simulink model "Copy_of_HIL_Serial"  (R2020a)
settings: Solver=ode4  StartTime=0.0  StopTime=inf  FixedStep=0.01  RelTol=1e-3  EnableMultiTasking=on
values from neighbouring files (symbols this model uses):
  Ue = [0.0416; -0.0703; 0; 0]    [equilibrium.m]    (also in start.m = [0.0416; -0.0703;      0;      0])
undefined symbols (not defined in the file or in its folder): LF, serial
libraries: instrumentlib x3
settings Model: PauseTimes=29  Creator=Marcelo Henrique  LastModifiedBy=waldene
settings SolverCC: AlgebraicLoopSolver=LineSearch
settings DataIOCC: LimitDataPoints=on  SaveFormat=Array  ReturnWorkspaceOutputs=off
settings OptimizationCC: LifeSpan=inf
settings DebuggingCC: AlgebraicLoopMsg=none  UnderspecifiedInitializationDetection=Classic  MergeDetectMultiDrivingBlocksExec=none  StateNameClashWarn=warning  SFUnexpectedBacktrackingDiag=warning  SFNoUnconditionalDefaultTransitionDiag=warning  ArithmeticOperatorsInVariantConditions=warning
settings HardwareCC: ProdBitPerPointer=32  ProdBitPerSizeT=32  ProdBitPerPtrDiffT=32  ProdLargestAtomicFloat=None  ProdIntDivRoundTo=Undefined  ProdEndianess=Unspecified  ProdWordSize=32  ProdHWDeviceType=32-bit Generic
settings ModelReferenceCC: PropagateSignalLabelsOutOfModel=off
settings SFSimCC: SimUseLocalCustomCode=off  CustomCodeUndefinedFunction=UseInterfaceOnly
settings RTWCC: RTWUseLocalCustomCode=off
settings CodeAppCC: StateflowObjectComments=on
settings GRTTargetCC: TargetLangStandard=C89/C90 (ANSI)
settings ConfigComp: CovMetricSettings=dw  CovHtmlReporting=on  CovSaveCumulativeToWorkspaceVar=on  CovSaveSingleToWorkspaceVar=on  CovExternalEMLEnable=off

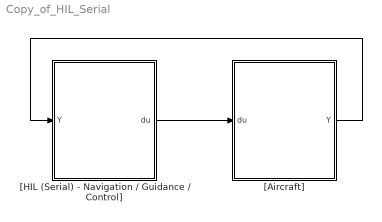
== system Copy_of_HIL_Serial ==
  "[Aircraft]" : Subsystem
  "[HIL (Serial) - Navigation / Guidance / Control]" : Subsystem
  wires:
  "[Aircraft]"/1(Y) -> "[HIL (Serial) - Navigation / Guidance / Control]"/1(Y)
  "[HIL (Serial) - Navigation / Guidance / Control]"/1(du) -> "[Aircraft]"/1(du)

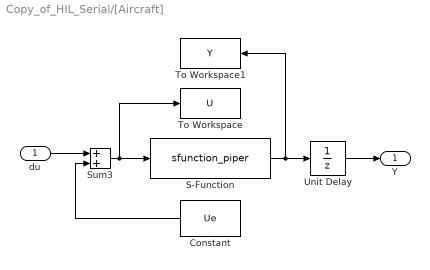
== system Copy_of_HIL_Serial/[Aircraft] ==
  du : Inport
  Constant : Constant  Value=Ue
  S-Function : S-Function  FunctionName=sfunction_piper  Parameters=par_gen,par_aero,par_prop, Xe  SFunctionDeploymentMode=off  EnableBusSupport=off
  Sum3 : Sum
  To Workspace : ToWorkspace  VariableName=U  SaveFormat=Timeseries  SampleTime=-1
  To Workspace1 : ToWorkspace  VariableName=Y  SaveFormat=Timeseries  SampleTime=-1
  Unit Delay : UnitDelay  SampleTime=-1  HasFrameUpgradeWarning=on
  Y : Outport
  wires:
  du/1 -> Sum3/1
  S-Function/1 -> To Workspace1/1, Unit Delay/1
  Constant/1 -> Sum3/2
  Sum3/1 -> To Workspace/1, S-Function/1
  Unit Delay/1 -> Y/1

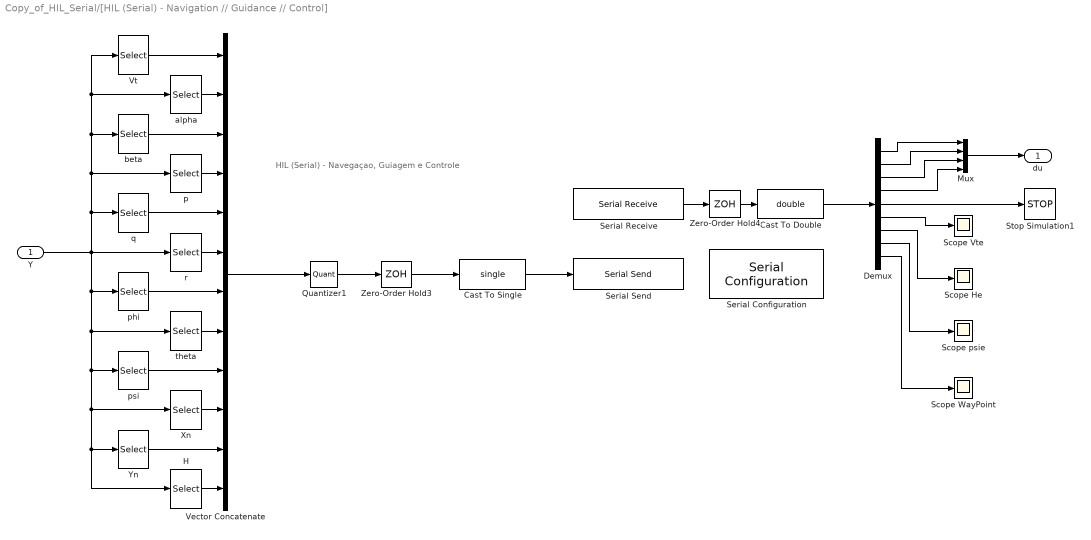
== system Copy_of_HIL_Serial/[HIL (Serial) - Navigation // Guidance // Control] ==
  note: HIL (Serial) - Navegaçao, Guiagem e Controle
  Y : Inport
  Cast To Double : DataTypeConversion  OutDataTypeStr=double
  Cast To Single : DataTypeConversion  OutDataTypeStr=single
  Demux : Demux  Outputs=9
  H : Selector  InputPortWidth=12  IndexOptions=Index vector (dialog)  Indices=[12]  OutputSizes=1
  Mux : Mux
  Quantizer1 : Quantizer  QuantizationInterval=0.01
  Scope He : Scope
  Scope Vte : Scope
  Scope WayPoint : Scope
  Scope psie : Scope
  Serial Configuration : instrumentlib/Serial Configuration  Priority=-200000  ComPortMenu=<Please select a port...>  ComPort=/dev/ttyUSB0  ObjConstructor=serial('/dev/ttyUSB0');  BaudRate=115200  DataBits=8  Parity=none  StopBits=1  FlowControl=none  Timeout=10  ByteOrder=LittleEndian
  Serial Receive : instrumentlib/Serial Receive  ComPortMenu=<Please select a port...>  ComPort=/dev/ttyUSB0  ObjConstructor=serial('/dev/ttyUSB0');  Header=A  Terminator=LF ('\n')  DataSize="[1  9]"  DataType=single  EnableBlockingMode=on  ActionDataUnavailable=Output last received value  CustomValue=0  SampleTime=0.01
  Serial Send : instrumentlib/Serial Send  ComPortMenu=<Please select a port...>  ComPort=/dev/ttyUSB0  ObjConstructor=serial('/dev/ttyUSB0');  Header=W  Terminator=<none>  EnableBlockingMode=on
  Stop Simulation1 : Stop
  Vector Concatenate : Concatenate  NumInputs=12
  Vt : Selector  InputPortWidth=12  IndexOptions=Index vector (dialog)  Indices=[1]  OutputSizes=1
  Xn : Selector  InputPortWidth=12  IndexOptions=Index vector (dialog)  Indices=[10]  OutputSizes=1
  Yn : Selector  InputPortWidth=12  IndexOptions=Index vector (dialog)  Indices=[11]  OutputSizes=1
  Zero-Order Hold3 : ZeroOrderHold  SampleTime=.01
  Zero-Order Hold4 : ZeroOrderHold  SampleTime=.01
  alpha : Selector  InputPortWidth=12  IndexOptions=Index vector (dialog)  Indices=[2]  OutputSizes=1
  beta : Selector  InputPortWidth=12  IndexOptions=Index vector (dialog)  Indices=[3]  OutputSizes=1
  p : Selector  InputPortWidth=12  IndexOptions=Index vector (dialog)  Indices=[4]  OutputSizes=1
  phi : Selector  InputPortWidth=12  IndexOptions=Index vector (dialog)  Indices=[7]  OutputSizes=1
  psi : Selector  InputPortWidth=12  IndexOptions=Index vector (dialog)  Indices=[9]  OutputSizes=1
  q : Selector  InputPortWidth=12  IndexOptions=Index vector (dialog)  Indices=[5]  OutputSizes=1
  r : Selector  InputPortWidth=12  IndexOptions=Index vector (dialog)  Indices=[6]  OutputSizes=1
  theta : Selector  InputPortWidth=12  IndexOptions=Index vector (dialog)  Indices=[8]  OutputSizes=1
  du : Outport
  wires:
  Zero-Order Hold3/1 -> Cast To Single/1
  Vector Concatenate/1 -> Quantizer1/1
  Serial Receive/1 -> Zero-Order Hold4/1
  Cast To Single/1 -> Serial Send/1
  Quantizer1/1 -> Zero-Order Hold3/1
  Zero-Order Hold4/1 -> Cast To Double/1
  Y/1 -> H/1, Yn/1, Xn/1, psi/1, theta/1, phi/1, r/1, Vt/1, alpha/1, beta/1, p/1, q/1
  Vt/1 -> Vector Concatenate/1
  alpha/1 -> Vector Concatenate/2
  beta/1 -> Vector Concatenate/3
  p/1 -> Vector Concatenate/4
  q/1 -> Vector Concatenate/5
  r/1 -> Vector Concatenate/6
  phi/1 -> Vector Concatenate/7
  theta/1 -> Vector Concatenate/8
  psi/1 -> Vector Concatenate/9
  Xn/1 -> Vector Concatenate/10
  Yn/1 -> Vector Concatenate/11
  H/1 -> Vector Concatenate/12
  Cast To Double/1 -> Demux/1
  Mux/1 -> du/1
  Demux/1 -> Mux/1
  Demux/2 -> Mux/2
  Demux/3 -> Mux/3
  Demux/4 -> Mux/4
  Demux/5 -> Stop Simulation1/1
  Demux/6 -> Scope Vte/1
  Demux/7 -> Scope He/1
  Demux/8 -> Scope psie/1
  Demux/9 -> Scope WayPoint/1
